simulink model "RL_sus_quarter_sim"  (R2025a)
settings: Solver=FixedStepAuto  StartTime=0.0  StopTime=20  FixedStep=0.001  RelTol=1e-3
model workspace (MAT data in the model file):
  G0 : Simulink.Parameter (value not decoded)
  Q_F : Simulink.Parameter (value not decoded)
  Q_dot_s : Simulink.Parameter (value not decoded)
  Q_dot_s_h : Simulink.Parameter (value not decoded)
  Q_dot_u : Simulink.Parameter (value not decoded)
  Q_flec : Simulink.Parameter (value not decoded)
  Q_flec_t : Simulink.Parameter (value not decoded)
  b_deflec : Simulink.Parameter (value not decoded)
  bump_height : Simulink.Parameter (value not decoded)
  bump_lenth : Simulink.Parameter (value not decoded)
  bump_start : Simulink.Parameter (value not decoded)
  f0 : Simulink.Parameter (value not decoded)
  kt : Simulink.Parameter (value not decoded)
  ms : Simulink.Parameter (value not decoded)
  n0 : Simulink.Parameter (value not decoded)
  n1 : Simulink.Parameter (value not decoded)
  omega_1 : Simulink.Parameter (value not decoded)
  omega_2 : Simulink.Parameter (value not decoded)
  omega_3 : Simulink.Parameter (value not decoded)
  omega_4 : Simulink.Parameter (value not decoded)
  ramp_height : Simulink.Parameter (value not decoded)
  ramp_lenth : Simulink.Parameter (value not decoded)
  ramp_start : Simulink.Parameter (value not decoded)
  sine_amp : Simulink.Parameter (value not decoded)
  sine_freq : Simulink.Parameter (value not decoded)
  u : Simulink.Parameter (value not decoded)
symbols that are objects in the model workspace (value not decoded): b_deflec, bump_height, bump_lenth, bump_start, f0, G0, kt, ms, n0, n1, omega_1, omega_2, omega_3, omega_4, Q_dot_s, Q_dot_s_h, Q_F, Q_flec, Q_flec_t, ramp_height, ramp_lenth, ramp_start, sine_amp, sine_freq
undefined symbols (not defined in the file): Ground, Hook, SH_ADD_new_as_as_xdef
libraries: fl_lib x250, nesl_utility x48, sharedTrackingLibrary x34, dspstat3 x18, simulink x3, deeplib x2, slpidlib x1
(part 5 of 12)

== system RL_sus_quarter_sim/Quarter_sys/Control/Y_1/SH_ADD_new_xdef_vs ==
  x_def : Inport
  v_def : Inport  Port=2
  v_s : Inport  Port=3
  a_s : Inport  Port=4
  a_def : Inport  Port=5
  2nd_FS_adef_vs : Subsystem
  ADD : Subsystem
  SH : Subsystem
  Scope : Scope
      settings: ActiveDisplayYMinimum=-69.71709  ActiveDisplayYMaximum=42.91727  DataLoggingVariableName=ScopeData19
  Scope1 : Scope
      settings: ActiveDisplayYMinimum=-36.33724  ActiveDisplayYMaximum=1.39762  DataLoggingVariableName=ScopeData21
  Switch1 : Switch  Criteria=u2 > Threshold  SaturateOnIntegerOverflow=off  InputSameDT=off
  F_sus : Outport
  wires:
  v_def/1 -> ADD/2(v_def), SH/1(v_def)
  x_def/1 -> Scope1/1, SH/3(x_def), ADD/1(x_def)
  ADD/1(F_sus1) -> Switch1/1
  SH/1(Out1) -> Switch1/3
  v_s/1 -> 2nd_FS_adef_vs/1(vs), SH/2(v_s)
  a_s/1 -> ADD/3(a_s)
  2nd_FS_adef_vs/1(FS2) -> Scope/1, Switch1/2
  Switch1/1 -> F_sus/1
  a_def/1 -> 2nd_FS_adef_vs/2(adef)

== system RL_sus_quarter_sim/Quarter_sys/Control/Y_1/Sky-Hook ==
  v_def : Inport
  v_s : Inport  Port=2
  x_def : Inport  Port=3
  Add : Sum
  Add1 : Sum
  Constant : Constant  Value=-1
  Constant1 : Constant
  Delta_C : Gain  Gain=500
  Gain : Gain  Gain=-1
  Lmbada_C : Constant  Value=1000
  Product : Product
  Product1 : Product
  Switch : Switch  Criteria=u2 > Threshold  SaturateOnIntegerOverflow=off  InputSameDT=off
  ks : Gain  Gain=-20000
  F_sus : Outport
  wires:
  Product/1 -> Switch/2
  v_s/1 -> Product/2
  v_def/1 -> Product1/1, Product/1
  Add/1 -> Product1/2
  Switch/1 -> Delta_C/1
  Product1/1 -> Gain/1
  Constant/1 -> Switch/3
  Constant1/1 -> Switch/1
  Lmbada_C/1 -> Add/2
  Delta_C/1 -> Add/1
  Gain/1 -> Add1/1
  Add1/1 -> F_sus/1
  ks/1 -> Add1/2
  x_def/1 -> ks/1

== system RL_sus_quarter_sim/Quarter_sys/Control/Y_1/decouple_Hinf ==
  x_def : Inport
  v_s : Inport  Port=2
  v_def : Inport  Port=3
  a_def : Inport  Port=4
  a_s : Inport  Port=5
  a_u : Inport  Port=6
  v_u : Inport  Port=7
  x_s : Inport  Port=8
  Add : Sum  Inputs=+-
  Add1 : Sum  Inputs=--
  Add2 : Sum
  Add3 : Sum
  Constant : Constant  Value=[10,10]  VectorParams1D=off
  Gain : Gain  Gain=-1
  Gain1 : Gain  Gain=20000
  Gain2 : Gain  Gain=1500
  Mux : Mux  Inputs=2
  Product : Product  Multiplication=Matrix(*)
  cs : Gain  Gain=-1000
  ks : Gain  Gain=-20000
  ms : Gain  Gain=400
  F_sus : Outport
  wires:
  Add1/1 -> Add/2  "alpha"
  Add/1 -> Add3/1
  Gain/1 -> ms/1  "v"
  Gain1/1 -> Add1/1
  Gain2/1 -> Add1/2
  ms/1 -> Add/1
  Add2/1 -> Add3/2  "passive"
  ks/1 -> Add2/1
  x_def/1 -> Mux/1, ks/1, Gain1/1
  v_def/1 -> cs/1, Gain2/1, Mux/2
  cs/1 -> Add2/2
  Add3/1 -> F_sus/1
  Constant/1 -> Product/1
  Product/1 -> Gain/1
  Mux/1 -> Product/2

== system RL_sus_quarter_sim/Quarter_sys/Control/Y_1/decouple_simple ==
  x_def : Inport
  v_s : Inport  Port=2
  v_def : Inport  Port=3
  a_def : Inport  Port=4
  a_s : Inport  Port=5
  a_u : Inport  Port=6
  v_u : Inport  Port=7
  x_s : Inport  Port=8
  x_u : Inport  Port=9
  Add : Sum  Inputs=+-
  Add1 : Sum  Inputs=--
  Add2 : Sum
  Add3 : Sum
  Gain1 : Gain  Gain=20000
  Gain2 : Gain  Gain=1500
  Gain3 : Gain  Gain=(-kt+100)/ms
  Gain4 : Gain  Gain=10/ms
  ms : Gain  Gain=400
  passive : Subsystem
  F_sus : Outport
  wires:
  Add3/1 -> F_sus/1
  v_def/1 -> passive/2(In2), Gain2/1  "vdef"
  x_def/1 -> Gain1/1, passive/1(In1)  "xdef"
  ms/1 -> Add/1
  Gain2/1 -> Add1/2
  Gain1/1 -> Add1/1
  Add2/1 -> ms/1  "v"
  Add/1 -> Add3/1
  Add1/1 -> Add/2  "alpha"
  passive/1(passive) -> Add3/2
  x_u/1 -> Gain3/1
  v_u/1 -> Gain4/1
  Gain3/1 -> Add2/1
  Gain4/1 -> Add2/2

== system RL_sus_quarter_sim/Quarter_sys/Control/Y_1/freq semi ==
  x_def : Inport
  v_def : Inport  Port=2
  a_def : Inport  Port=3
  a_s : Inport  Port=4
  v_s : Inport  Port=5
  a_u : Inport  Port=6
  ADD : Subsystem
  Multiport Switch : MultiPortSwitch  SaturateOnIntegerOverflow=off  InputSameDT=off
  Multiport Switch1 : MultiPortSwitch  Commented=on  SaturateOnIntegerOverflow=off  InputSameDT=off
  SH : Subsystem
  Scope : Scope
      settings: ActiveDisplayYMinimum=1.00019  ActiveDisplayYMaximum=3.05477  DataLoggingVariableName=ScopeData6
  Scope1 : Scope  Commented=on  NumInputPorts=2
      settings: ActiveDisplayYMinimum=-22.33402  ActiveDisplayYMaximum=17.66511  DataLoggingVariableName=ScopeData5
  Scope2 : Scope  Commented=on
      settings: ActiveDisplayYMinimum=-1695.55215  ActiveDisplayYMaximum=1442.87782  DataLoggingVariableName=ScopeData6
  Scope3 : Scope  Commented=on
      settings: ActiveDisplayYMinimum=-838.91856  ActiveDisplayYMaximum=95.65649  DataLoggingVariableName=ScopeData7
  Subsystem : Subsystem
  Subsystem1 : Subsystem
  Subsystem2 : Subsystem  Commented=on
  Subsystem3 : Subsystem  Commented=on
  Switch : Switch  Commented=on  Criteria=u2 > Threshold  SaturateOnIntegerOverflow=off  InputSameDT=off
  To Workspace : ToWorkspace  VariableName=FS_result  SampleTime=-1
  F_sus : Outport
  wires:
  v_s/1 -> Subsystem/1(vs), SH/2(v_s)
  a_s/1 -> ADD/3(a_s), Subsystem/3(as)
  v_def/1 -> ADD/2(v_def), SH/1(v_def), Subsystem1/1(v_def), Subsystem2/1(v_def), Subsystem3/1(v_def)
  x_def/1 -> Subsystem2/2(x_def), Subsystem3/2(x_def), Subsystem1/2(x_def), SH/3(x_def), ADD/1(x_def)
  Subsystem1/1(Out1) -> Multiport Switch1/4, Switch/1, Multiport Switch/4
  SH/1(Out1) -> Multiport Switch/2
  ADD/1(F_sus1) -> Multiport Switch/3
  Multiport Switch/1 -> F_sus/1
  Multiport Switch1/1 -> ?
  Subsystem2/1(Out1) -> Multiport Switch1/2, Switch/3
  Subsystem3/1(Out1) -> Multiport Switch1/3
  Switch/1 -> Scope2/1
  Subsystem/2(FS_1) -> Scope1/1, Scope3/1, Switch/2
  a_u/1 -> Subsystem/2(au)
  Subsystem/3(FS_2) -> Scope1/2
  Subsystem/1(Select) -> Multiport Switch1/1, Scope/1, To Workspace/1, Multiport Switch/1

== system RL_sus_quarter_sim/Quarter_sys/Control/Y_1/imp_force_RL_model ==
  x_def : Inport
  v_s : Inport  Port=2
  v_def : Inport  Port=3
  a_def : Inport  Port=4
  a_s : Inport  Port=5
  Add2 : Sum  Inputs=+++
  Add3 : Sum
  Gain : Gain  Gain=1000
  Gain1 : Gain  Gain=1/5
  Gain2 : Gain  Gain=1/0.3
  Gain3 : Gain  Gain=1/0.03
  Mux : Mux
  Predict1 : deeplib/Predict  Network=Network from MAT-file  NetworkFunction=squeezenet  NetworkFilePath=D:\Project\GOPS\mdl\RL_model\TD3_270374_opt.mat  MiniBatchSize=128  InputDataFormats={ 'input_1', 'UU' }  Predictions=on  Activations={}  ForceInterpretedSim=off  EnableDLNetwork=on  LastKnownNetworkFilePath='D:\Project\GOPS\mdl\RL_model\TD3_270374_opt.mat'  LastKnownNetworkTimeStamp=739967.681944444426335394382476806640625
  Rate Transition : RateTransition  OutPortSampleTime=0.01
  Reshape : Reshape  OutputDimensionality=Row vector (2-D)
  Reshape2 : Reshape
  Saturation : Saturate  UpperLimit=1000  LowerLimit=-1000
  Subsystem : Subsystem
  bkkcc : Subsystem
  cs1 : Gain  Gain=-1000
  ks1 : Gain  Gain=-20000
  F_sus : Outport
  F_ctr : Outport  Port=2
  wires:
  Gain2/1 -> Mux/4
  Rate Transition/1 -> Predict1/1
  Reshape2/1 -> Gain/1
  Gain/1 -> Saturation/1
  Gain3/1 -> Mux/3
  Gain1/1 -> Mux/1
  Reshape/1 -> Rate Transition/1
  Mux/1 -> Reshape/1
  Predict1/1 -> Reshape2/1
  v_def/1 -> bkkcc/1(v_def), cs1/1, Gain2/1
  a_def/1 -> bkkcc/3(a_def)
  cs1/1 -> Add2/2  "F_damper"
  ks1/1 -> Add2/1
  x_def/1 -> ks1/1, bkkcc/2(x_def), Gain3/1
  Subsystem/1(Out1) -> bkkcc/4(param_ctr)
  bkkcc/1(F_bkkcc) -> Add2/3
  v_s/1 -> Subsystem/1(v_s), Mux/2
  Add2/1 -> Add3/2
  Add3/1 -> F_sus/1
  a_s/1 -> Gain1/1
  Saturation/1 -> Add3/1, F_ctr/1

== system RL_sus_quarter_sim/Quarter_sys/Control/Y_1/lqr ==
  x_s : Inport
  v_s : Inport  Port=2
  x_def : Inport  Port=3
  v_def : Inport  Port=4
  Add : Sum  Inputs=+-
  Add1 : Sum  Inputs=+++
  Add2 : Sum  Inputs=+-
  Gain : Gain  Gain=-1
  K : Constant  Value="[-824.335747522357\t31.6227766016762\t-0.106412814889091\t-3.16537773169978]"
  Mux : Mux
  Product : Product  Multiplication=Matrix(*)
  To Workspace : ToWorkspace  VariableName=F_if_imp  SampleTime=-1
  cs : Gain  Gain=-1000
  ks : Gain  Gain=-20000
  F_sus : Outport
  wires:
  v_def/1 -> Add2/2, cs/1
  v_s/1 -> Add2/1, Mux/2  "vs"
  x_s/1 -> Add/1, ks/1, Mux/1  "xs"
  Add1/1 -> F_sus/1
  ks/1 -> Add1/1
  cs/1 -> Add1/2  "F_damper"
  x_def/1 -> Add/2
  Add/1 -> Mux/3  "xu"
  Add2/1 -> Mux/4  "vu"
  K/1 -> Product/2
  Mux/1 -> Product/1
  Product/1 -> Gain/1
  Gain/1 -> Add1/3, To Workspace/1

== system RL_sus_quarter_sim/Quarter_sys/Passive/Y_1/P_0 ==
  x_def : Inport
  v_def : Inport  Port=2
  a_def : Inport  Port=3
  Add1 : Sum
  Ideal Force Sensor : fl_lib/Mechanical/Mechanical Sensors/Ideal Force Sensor
  Ideal Translational Velocity Source : fl_lib/Mechanical/Mechanical Sources/Ideal Translational Velocity Source
  Mechanical Translational Reference : fl_lib/Mechanical/Translational Elements/Mechanical Translational Reference
  Mechanical Translational Reference1 : fl_lib/Mechanical/Translational Elements/Mechanical Translational Reference
  PS-Simulink Converter : nesl_utility/PS-Simulink Converter  PhysicalDomain=network_engine_domain  SubClassName=ps_output  LeftPortType=input  RightPortType=output  PseudoPeriodic=off  Frequencies=[]  VectorFormat=inherit  Unit=inherit  AffineConversion=off
  Scope : Scope  NumInputPorts=2
      settings: ActiveDisplayYMinimum=-2784.63973  ActiveDisplayYMaximum=3155.95467
  Simulink-PS Converter : nesl_utility/Simulink-PS Converter  PhysicalDomain=network_engine_domain  SubClassName=ps_input  LeftPortType=input  RightPortType=output  PseudoPeriodic=off  Frequencies=[]  NoiseDistribution=none  NoiseParameters=[]  Unit=1  AffineConversion=off  FilteringAndDerivatives=provide  SimscapeFilterOrder=1  InputFilterTimeConstant=0.001  UdotUserProvided=0
  Solver Configuration : nesl_utility/Solver Configuration  PhysicalDomain=network_engine_domain  SubClassName=solver  LeftPortType=input  RightPortType=generic  Tones=[]  Harmonics=[]  SimulateNoise=off  Profile=off  UseLocalSampling=off  EnableSwitchedLinearOptims=on  FrequencyDomain=off  UseCCode=off  RelTol=0.001  AbsTol=0.001  MinStep=1e-09  ToWorkspace=off  RevertToSquareIcSolve=off  NumHomotopyIterations=100  PhasorMode=off  PhasorModeNumHarmonics=1  ConsistencySolver=NEWTON_XTOL_AFTER_FTOL  IndexReductionMethod=DerivativeReplacement  DoDC=off  ResidualTolerance=1e-09  ConsistencyTolSource=GLOBAL  ConsistencyAbsTol=0.001  ConsistencyRelTol=0.001  ConsistencyTolFactor=0.001  UseLocalSolver=off  LocalSolverChoice=NE_BACKWARD_EULER_ADVANCER  ResolveIndetEquations=on  FunctionEvalNumThread=1  LocalSolverSampleTime=0.001  DoFixedCost=off  MaxNonlinIter=3  MaxModeIter=2  ComputeImpulses=off  ImpulseIterations=2  LinearAlgebra=auto  LinearAlgebraNumThread=0  EquationFormulation=NE_TIME_EF  DelaysMemoryBudget=1024  AutomaticFiltering=on  FilteringTimeConstant=0.001  PartitionStorageMethod=AS_NEEDED  PartitionMemoryBudget=1024  PartitionMethod=ROBUST  MultibodyUseLocalSolver=off  MultibodyLocalSolverChoice=ODE1  MultibodyLocalSolverSampleTime=0.001
  Subsystem : Subsystem  Variant=on  VariantControlMode=label  VariantControl=Subsystem  LabelModeActiveChoice=p0_k6
  cs : Gain  Gain=-2000
  ks : Gain  Gain=-200000
  F_sus : Outport
  wires:
  x_def/1 -> ks/1
  cs/1 -> Add1/2
  ks/1 -> Add1/1
  v_def/1 -> Simulink-PS Converter/1, cs/1
  PS-Simulink Converter/1 -> F_sus/1, Scope/1
  connections:
  Mechanical Translational Reference1/LConn1 -- Solver Configuration/RConn1 -- Ideal Translational Velocity Source/LConn1
  Simulink-PS Converter/RConn1 -- Ideal Translational Velocity Source/RConn1
  Ideal Force Sensor/RConn1 -- Mechanical Translational Reference/LConn1
  PS-Simulink Converter/LConn1 -- Ideal Force Sensor/RConn2
  Subsystem/LConn1 -- Ideal Translational Velocity Source/RConn2
  Subsystem/RConn1 -- Ideal Force Sensor/LConn1

== system RL_sus_quarter_sim/Quarter_sys/Passive/Y_1/P_1 ==
  x_def : Inport
  v_def : Inport  Port=2
  a_def : Inport  Port=3
  Add1 : Sum
  Ideal Force Sensor : fl_lib/Mechanical/Mechanical Sensors/Ideal Force Sensor
  Ideal Translational Velocity Source : fl_lib/Mechanical/Mechanical Sources/Ideal Translational Velocity Source
  Mechanical Translational Reference : fl_lib/Mechanical/Translational Elements/Mechanical Translational Reference
  Mechanical Translational Reference1 : fl_lib/Mechanical/Translational Elements/Mechanical Translational Reference
  PS-Simulink Converter : nesl_utility/PS-Simulink Converter  PhysicalDomain=network_engine_domain  SubClassName=ps_output  LeftPortType=input  RightPortType=output  PseudoPeriodic=off  Frequencies=[]  VectorFormat=inherit  Unit=inherit  AffineConversion=off
  Scope : Scope  NumInputPorts=2
      settings: ActiveDisplayYMinimum=-2784.63973  ActiveDisplayYMaximum=3155.95467
  Simulink-PS Converter : nesl_utility/Simulink-PS Converter  PhysicalDomain=network_engine_domain  SubClassName=ps_input  LeftPortType=input  RightPortType=output  PseudoPeriodic=off  Frequencies=[]  NoiseDistribution=none  NoiseParameters=[]  Unit=1  AffineConversion=off  FilteringAndDerivatives=provide  SimscapeFilterOrder=1  InputFilterTimeConstant=0.001  UdotUserProvided=1
  Solver Configuration : nesl_utility/Solver Configuration  PhysicalDomain=network_engine_domain  SubClassName=solver  LeftPortType=input  RightPortType=generic  Tones=[]  Harmonics=[]  SimulateNoise=off  Profile=off  UseLocalSampling=off  EnableSwitchedLinearOptims=on  FrequencyDomain=off  UseCCode=off  RelTol=0.001  AbsTol=0.001  MinStep=1e-09  ToWorkspace=off  RevertToSquareIcSolve=off  NumHomotopyIterations=100  PhasorMode=off  PhasorModeNumHarmonics=1  ConsistencySolver=NEWTON_XTOL_AFTER_FTOL  IndexReductionMethod=DerivativeReplacement  DoDC=off  ResidualTolerance=1e-09  ConsistencyTolSource=GLOBAL  ConsistencyAbsTol=0.001  ConsistencyRelTol=0.001  ConsistencyTolFactor=0.001  UseLocalSolver=off  LocalSolverChoice=NE_BACKWARD_EULER_ADVANCER  ResolveIndetEquations=on  FunctionEvalNumThread=1  LocalSolverSampleTime=0.001  DoFixedCost=off  MaxNonlinIter=3  MaxModeIter=2  ComputeImpulses=off  ImpulseIterations=2  LinearAlgebra=auto  LinearAlgebraNumThread=0  EquationFormulation=NE_TIME_EF  DelaysMemoryBudget=1024  AutomaticFiltering=on  FilteringTimeConstant=0.001  PartitionStorageMethod=AS_NEEDED  PartitionMemoryBudget=1024  PartitionMethod=ROBUST  MultibodyUseLocalSolver=off  MultibodyLocalSolverChoice=ODE1  MultibodyLocalSolverSampleTime=0.001
  Subsystem : Subsystem  Variant=on  VariantControlMode=label  VariantControl=Subsystem  LabelModeActiveChoice=p1_k3
  cs : Gain  Gain=-2000
  ks : Gain  Gain=-200000
  F_sus : Outport
  wires:
  PS-Simulink Converter/1 -> F_sus/1, Scope/1
  v_def/1 -> cs/1, Simulink-PS Converter/1
  ks/1 -> Add1/1
  cs/1 -> Add1/2
  x_def/1 -> ks/1
  a_def/1 -> Simulink-PS Converter/2
  connections:
  Subsystem/RConn1 -- Ideal Force Sensor/LConn1
  Subsystem/LConn1 -- Ideal Translational Velocity Source/RConn2
  PS-Simulink Converter/LConn1 -- Ideal Force Sensor/RConn2
  Ideal Force Sensor/RConn1 -- Mechanical Translational Reference/LConn1
  Simulink-PS Converter/RConn1 -- Ideal Translational Velocity Source/RConn1
  Solver Configuration/RConn1 -- Mechanical Translational Reference1/LConn1 -- Ideal Translational Velocity Source/LConn1

== system RL_sus_quarter_sim/Quarter_sys/Passive/Y_1/P_test ==
  x_def : Inport
  v_def : Inport  Port=2
  a_def : Inport  Port=3
  Add : Sum  Inputs=+-
  Add1 : Sum
  Ideal Force Sensor : fl_lib/Mechanical/Mechanical Sensors/Ideal Force Sensor
  Ideal Translational Velocity Source : fl_lib/Mechanical/Mechanical Sources/Ideal Translational Velocity Source
  Integrator : Integrator
  Mechanical Translational Reference : fl_lib/Mechanical/Translational Elements/Mechanical Translational Reference
  Mechanical Translational Reference1 : fl_lib/Mechanical/Translational Elements/Mechanical Translational Reference
  PS-Simulink Converter : nesl_utility/PS-Simulink Converter  PhysicalDomain=network_engine_domain  SubClassName=ps_output  LeftPortType=input  RightPortType=output  PseudoPeriodic=off  Frequencies=[]  VectorFormat=inherit  Unit=inherit  AffineConversion=off
  Scope : Scope  NumInputPorts=2
      settings: ActiveDisplayYMinimum=-1294.98501  ActiveDisplayYMaximum=1379.176
  Simulink-PS Converter : nesl_utility/Simulink-PS Converter  PhysicalDomain=network_engine_domain  SubClassName=ps_input  LeftPortType=input  RightPortType=output  PseudoPeriodic=off  Frequencies=[]  NoiseDistribution=none  NoiseParameters=[]  Unit=1  AffineConversion=off  FilteringAndDerivatives=provide  SimscapeFilterOrder=1  InputFilterTimeConstant=0.001  UdotUserProvided=1
  Solver Configuration : nesl_utility/Solver Configuration  PhysicalDomain=network_engine_domain  SubClassName=solver  LeftPortType=input  RightPortType=generic  Tones=[]  Harmonics=[]  SimulateNoise=off  Profile=off  UseLocalSampling=off  EnableSwitchedLinearOptims=on  FrequencyDomain=off  UseCCode=off  RelTol=0.001  AbsTol=0.001  MinStep=1e-09  ToWorkspace=off  RevertToSquareIcSolve=off  NumHomotopyIterations=100  PhasorMode=off  PhasorModeNumHarmonics=1  ConsistencySolver=NEWTON_XTOL_AFTER_FTOL  IndexReductionMethod=DerivativeReplacement  DoDC=off  ResidualTolerance=1e-09  ConsistencyTolSource=GLOBAL  ConsistencyAbsTol=0.001  ConsistencyRelTol=0.001  ConsistencyTolFactor=0.001  UseLocalSolver=off  LocalSolverChoice=NE_BACKWARD_EULER_ADVANCER  ResolveIndetEquations=on  FunctionEvalNumThread=1  LocalSolverSampleTime=0.001  DoFixedCost=off  MaxNonlinIter=3  MaxModeIter=2  ComputeImpulses=off  ImpulseIterations=2  LinearAlgebra=auto  LinearAlgebraNumThread=0  EquationFormulation=NE_TIME_EF  DelaysMemoryBudget=1024  AutomaticFiltering=on  FilteringTimeConstant=0.001  PartitionStorageMethod=AS_NEEDED  PartitionMemoryBudget=1024  PartitionMethod=ROBUST  MultibodyUseLocalSolver=off  MultibodyLocalSolverChoice=ODE1  MultibodyLocalSolverSampleTime=0.001
  Subsystem : Subsystem  Commented=on  Variant=on  VariantControlMode=label  VariantControl=Subsystem  LabelModeActiveChoice=p1_k3
  Translational Damper : fl_lib/Mechanical/Translational Elements/Translational Damper  D=2000 N*s/m  v_specify=off  v_priority=None  v=0 m/s  v_nominal_specify=off  v_nominal_value=1  v_nominal_unit=m/s  f_specify=off  f_priority=None  f=0 N  f_nominal_specify=off  f_nominal_value=1  f_nominal_unit=N
  Translational Spring1 : fl_lib/Mechanical/Translational Elements/Translational Spring  spr_rate=200000 N/m  v_specify=off  v_priority=None  v=0 m/s  v_nominal_specify=off  v_nominal_value=1  v_nominal_unit=m/s  f_specify=off  f_priority=None  f=0 N  f_nominal_specify=off  f_nominal_value=1  f_nominal_unit=N  x_specify=off  x_priority=High  x=0 m  x_nominal_specify=off  x_nominal_value=1  x_nominal_unit=m
  Translational Spring2 : fl_lib/Mechanical/Translational Elements/Translational Spring  spr_rate=20000 N/m  v_specify=off  v_priority=None  v=0 m/s  v_nominal_specify=off  v_nominal_value=1  v_nominal_unit=m/s  f_specify=off  f_priority=None  f=0 N  f_nominal_specify=off  f_nominal_value=1  f_nominal_unit=N  x_specify=off  x_priority=High  x=0 m  x_nominal_specify=off  x_nominal_value=1  x_nominal_unit=m
  cs : Gain  Gain=-2000
  cs1 : Gain  Gain=20000/2000
  ks : Gain  Gain=-20000
  ks1 : Gain  Gain=-20000
  F_sus : Outport
  wires:
  a_def/1 -> Simulink-PS Converter/2
  x_def/1 -> ks/1
  cs/1 -> Add1/2
  ks/1 -> Add1/1
  v_def/1 -> ks1/1, Simulink-PS Converter/1, cs/1
  PS-Simulink Converter/1 -> Scope/1, F_sus/1
  Integrator/1 -> cs1/1, Scope/2
  ks1/1 -> Add/1
  Add/1 -> Integrator/1
  cs1/1 -> Add/2
  connections:
  Ideal Translational Velocity Source/LConn1 -- Mechanical Translational Reference1/LConn1 -- Solver Configuration/RConn1
  Simulink-PS Converter/RConn1 -- Ideal Translational Velocity Source/RConn1
  Ideal Force Sensor/RConn1 -- Mechanical Translational Reference/LConn1
  PS-Simulink Converter/LConn1 -- Ideal Force Sensor/RConn2
  Subsystem/LConn1 -- Translational Spring2/LConn1 -- Translational Damper/LConn1 -- Ideal Translational Velocity Source/RConn2
  Subsystem/RConn1 -- Translational Spring2/RConn1 -- Translational Spring1/RConn1 -- Ideal Force Sensor/LConn1
  Translational Spring1/LConn1 -- Translational Damper/RConn1

== system RL_sus_quarter_sim/Quarter_sys/Passive/Y_1/Passive ==
  x_def : Inport
  v_def : Inport  Port=2
  a_def : Inport  Port=3
  Add1 : Sum
  cs : Gain  Gain=-7.5
  ks : Gain  Gain=-900
  F_sus : Outport
  wires:
  Add1/1 -> F_sus/1
  v_def/1 -> cs/1
  ks/1 -> Add1/1
  cs/1 -> Add1/2
  x_def/1 -> ks/1

== system RL_sus_quarter_sim/Quarter_sys/Passive/Y_1/Sky-Hook ==
  x_def : Inport
  v_def : Inport  Port=2
  a_def : Inport  Port=3
  Add : Sum  Inputs=+-
  Add1 : Sum
  Ideal Force Sensor : fl_lib/Mechanical/Mechanical Sensors/Ideal Force Sensor
  Ideal Translational Velocity Source : fl_lib/Mechanical/Mechanical Sources/Ideal Translational Velocity Source
  Integrator : Integrator
  Mechanical Translational Reference : fl_lib/Mechanical/Translational Elements/Mechanical Translational Reference
  Mechanical Translational Reference1 : fl_lib/Mechanical/Translational Elements/Mechanical Translational Reference
  PS-Simulink Converter : nesl_utility/PS-Simulink Converter  PhysicalDomain=network_engine_domain  SubClassName=ps_output  LeftPortType=input  RightPortType=output  PseudoPeriodic=off  Frequencies=[]  VectorFormat=inherit  Unit=inherit  AffineConversion=off
  Scope : Scope  NumInputPorts=2
      settings: ActiveDisplayYMinimum=-1294.98501  ActiveDisplayYMaximum=1379.176
  Simulink-PS Converter : nesl_utility/Simulink-PS Converter  PhysicalDomain=network_engine_domain  SubClassName=ps_input  LeftPortType=input  RightPortType=output  PseudoPeriodic=off  Frequencies=[]  NoiseDistribution=none  NoiseParameters=[]  Unit=1  AffineConversion=off  FilteringAndDerivatives=provide  SimscapeFilterOrder=1  InputFilterTimeConstant=0.001  UdotUserProvided=1
  Solver Configuration : nesl_utility/Solver Configuration  PhysicalDomain=network_engine_domain  SubClassName=solver  LeftPortType=input  RightPortType=generic  Tones=[]  Harmonics=[]  SimulateNoise=off  Profile=off  UseLocalSampling=off  EnableSwitchedLinearOptims=on  FrequencyDomain=off  UseCCode=off  RelTol=0.001  AbsTol=0.001  MinStep=1e-09  ToWorkspace=off  RevertToSquareIcSolve=off  NumHomotopyIterations=100  PhasorMode=off  PhasorModeNumHarmonics=1  ConsistencySolver=NEWTON_XTOL_AFTER_FTOL  IndexReductionMethod=DerivativeReplacement  DoDC=off  ResidualTolerance=1e-09  ConsistencyTolSource=GLOBAL  ConsistencyAbsTol=0.001  ConsistencyRelTol=0.001  ConsistencyTolFactor=0.001  UseLocalSolver=off  LocalSolverChoice=NE_BACKWARD_EULER_ADVANCER  ResolveIndetEquations=on  FunctionEvalNumThread=1  LocalSolverSampleTime=0.001  DoFixedCost=off  MaxNonlinIter=3  MaxModeIter=2  ComputeImpulses=off  ImpulseIterations=2  LinearAlgebra=auto  LinearAlgebraNumThread=0  EquationFormulation=NE_TIME_EF  DelaysMemoryBudget=1024  AutomaticFiltering=on  FilteringTimeConstant=0.001  PartitionStorageMethod=AS_NEEDED  PartitionMemoryBudget=1024  PartitionMethod=ROBUST  MultibodyUseLocalSolver=off  MultibodyLocalSolverChoice=ODE1  MultibodyLocalSolverSampleTime=0.001
  Subsystem : Subsystem  Commented=on  Variant=on  VariantControlMode=label  VariantControl=Subsystem  LabelModeActiveChoice=p1_k3
  Translational Damper : fl_lib/Mechanical/Translational Elements/Translational Damper  D=2000 N*s/m  v_specify=off  v_priority=None  v=0 m/s  v_nominal_specify=off  v_nominal_value=1  v_nominal_unit=m/s  f_specify=off  f_priority=None  f=0 N  f_nominal_specify=off  f_nominal_value=1  f_nominal_unit=N
  Translational Spring1 : fl_lib/Mechanical/Translational Elements/Translational Spring  spr_rate=200000 N/m  v_specify=off  v_priority=None  v=0 m/s  v_nominal_specify=off  v_nominal_value=1  v_nominal_unit=m/s  f_specify=off  f_priority=None  f=0 N  f_nominal_specify=off  f_nominal_value=1  f_nominal_unit=N  x_specify=off  x_priority=High  x=0 m  x_nominal_specify=off  x_nominal_value=1  x_nominal_unit=m
  Translational Spring2 : fl_lib/Mechanical/Translational Elements/Translational Spring  spr_rate=20000 N/m  v_specify=off  v_priority=None  v=0 m/s  v_nominal_specify=off  v_nominal_value=1  v_nominal_unit=m/s  f_specify=off  f_priority=None  f=0 N  f_nominal_specify=off  f_nominal_value=1  f_nominal_unit=N  x_specify=off  x_priority=High  x=0 m  x_nominal_specify=off  x_nominal_value=1  x_nominal_unit=m
  cs : Gain  Gain=-2000
  cs1 : Gain  Gain=20000/2000
  ks : Gain  Gain=-20000
  ks1 : Gain  Gain=-20000
  F_sus : Outport
  wires:
  cs1/1 -> Add/2
  Add/1 -> Integrator/1
  ks1/1 -> Add/1
  Integrator/1 -> Scope/2, cs1/1
  PS-Simulink Converter/1 -> F_sus/1, Scope/1
  v_def/1 -> cs/1, Simulink-PS Converter/1, ks1/1
  ks/1 -> Add1/1
  cs/1 -> Add1/2
  x_def/1 -> ks/1
  a_def/1 -> Simulink-PS Converter/2
  connections:
  Translational Spring1/LConn1 -- Translational Damper/RConn1
  Translational Spring2/RConn1 -- Translational Spring1/RConn1 -- Subsystem/RConn1 -- Ideal Force Sensor/LConn1
  Translational Spring2/LConn1 -- Translational Damper/LConn1 -- Subsystem/LConn1 -- Ideal Translational Velocity Source/RConn2
  PS-Simulink Converter/LConn1 -- Ideal Force Sensor/RConn2
  Ideal Force Sensor/RConn1 -- Mechanical Translational Reference/LConn1
  Simulink-PS Converter/RConn1 -- Ideal Translational Velocity Source/RConn1
  Solver Configuration/RConn1 -- Mechanical Translational Reference1/LConn1 -- Ideal Translational Velocity Source/LConn1

== system RL_sus_quarter_sim/road_profile/origin/road_profile/Bump ==
  Add : Sum
  Add1 : Sum  Inputs=+-
  Clock1 : Clock
  Constant : Constant  Value=bump_height
  Constant1 : Constant  Value=0
  Constant2 : Constant  Value=u
  Constant3 : Constant  Value=bump_start
  Constant4 : Constant  Value=bump_lenth
  Divide : Product  Inputs=*/
  Gain : Gain  Gain=1/3.6
  Product : Product
  Sine Wave1 : Sin  TimeSource=Use external signal  Amplitude=bump_height  Frequency=2*pi*1  Phase=-1/2*pi  SampleTime=0
  Switch : Switch  Criteria=u2 > Threshold  Threshold=bump_start  SaturateOnIntegerOverflow=off  InputSameDT=off
  Switch1 : Switch  Criteria=u2 > Threshold  Threshold=bump_lenth+bump_start  SaturateOnIntegerOverflow=off  InputSameDT=off
  Zr : Outport  VectorParamsAs1DForOutWhenUnconnected=off
  wires:
  Divide/1 -> Sine Wave1/1
  Constant/1 -> Add/2
  Add/1 -> Switch/1
  Constant4/1 -> Divide/2
  Add1/1 -> Divide/1
  Product/1 -> Gain/1
  Constant2/1 -> Product/1
  Constant3/1 -> Add1/2
  Constant1/1 -> Switch1/1, Switch/3
  Switch/1 -> Switch1/3
  Gain/1 -> Switch1/2, Switch/2, Add1/1
  Sine Wave1/1 -> Add/1
  Clock1/1 -> Product/2
  Switch1/1 -> Zr/1

== system RL_sus_quarter_sim/road_profile/origin/road_profile/Ramp ==
  Add : Sum
  Add1 : Sum  Inputs=+-
  Clock1 : Clock
  Constant : Constant  Value=ramp_height
  Constant1 : Constant  Value=0
  Constant2 : Constant  Value=u
  Constant3 : Constant  Value=ramp_start
  Constant4 : Constant  Value=ramp_lenth
  Constant5 : Constant  Value=ramp_height
  Divide : Product  Inputs=*/
  Gain : Gain  Gain=1/3.6
  Gain1 : Gain  Gain=2
  Gain2 : Gain  Gain=1/2
  Product : Product
  Sine Wave1 : Sin  TimeSource=Use external signal  Amplitude=bump_height/2  Frequency=2*pi*1  Phase=-1/2*pi  SampleTime=0
  Switch : Switch  Criteria=u2 > Threshold  Threshold=bump_start  SaturateOnIntegerOverflow=off  InputSameDT=off
  Switch1 : Switch  Criteria=u2 > Threshold  Threshold=ramp_lenth+ramp_start  SaturateOnIntegerOverflow=off  InputSameDT=off
  Zr : Outport  VectorParamsAs1DForOutWhenUnconnected=off
  wires:
  Switch1/1 -> Zr/1
  Clock1/1 -> Product/2
  Sine Wave1/1 -> Add/1
  Gain/1 -> Add1/1, Switch/2, Switch1/2
  Switch/1 -> Switch1/3
  Constant1/1 -> Switch/3
  Constant3/1 -> Add1/2
  Constant2/1 -> Product/1
  Product/1 -> Gain/1
  Add1/1 -> Divide/1
  Constant4/1 -> Gain1/1
  Add/1 -> Switch/1
  Constant/1 -> Gain2/1
  Divide/1 -> Sine Wave1/1
  Gain1/1 -> Divide/2
  Constant5/1 -> Switch1/1
  Gain2/1 -> Add/2

== system RL_sus_quarter_sim/road_profile/origin/road_profile/Random ==
  Add : Sum
  Gain : Gain  Gain=2*n0*pi*sqrt(G0*u)
  Gain1 : Gain  Gain=-2*pi*u*n1
  Integrator : Integrator
  WhiteNoise : simulink/Sources/Band-Limited White Noise  Cov=[0.5]  Ts=1/10/u  seed=[24553]
  Zr : Outport  VectorParamsAs1DForOutWhenUnconnected=off
  wires:
  Gain1/1 -> Add/2
  Add/1 -> Integrator/1
  WhiteNoise/1 -> Gain/1
  Integrator/1 -> Zr/1, Gain1/1
  Gain/1 -> Add/1

== system RL_sus_quarter_sim/road_profile/origin/road_profile/Sine ==
  Add : Sum
  Add1 : Sum
  Clock : Clock
  Gain : Gain  Gain=2*pi
  Scope : Scope  NumInputPorts=2
      settings: ActiveDisplayYMinimum=-0.00065  ActiveDisplayYMaximum=0.00585  DataLoggingVariableName=ScopeData2
  Sin : Trigonometry
  Sine Wave : Sin  Commented=on  Amplitude=sine_amp  Bias=sine_amp  Frequency=2*pi*sine_freq  Phase=-pi/2  SampleTime=0
  freq : Gain  Gain=9
  off-set : Constant
  phase : Constant  Value=-pi/2
  sine_amp : Gain  Gain=0.026/9
  Out1 : Outport
  wires:
  sine_amp/1 -> Out1/1, Scope/1
  Sin/1 -> Add/1
  Add/1 -> sine_amp/1
  off-set/1 -> Add/2
  phase/1 -> Add1/2
  Add1/1 -> Sin/1
  Gain/1 -> Add1/1
  freq/1 -> Gain/1
  Clock/1 -> freq/1
  Sine Wave/1 -> Scope/2

== system RL_sus_quarter_sim/road_profile/origin/road_profile/chirp ==
  note: 幅值
  note: 30hz
  note: f=t*0.2
  note: Frequency=0.2*t [Hz]
  note: x=sin(0.2*2pi*t*t)/(0.2*pi*t)
  Clock1 : Clock
  Constant1 : Constant  Value=0.001  SampleTime=0.001
  Constant2 : Constant
  Constant3 : Constant  Value=pi  SampleTime=0.001
  Divide4 : Product  Inputs=*/
  Divide5 : Product  Inputs=**
  Divide6 : Product  Inputs=**
  Divide7 : Product  Inputs=**
  Gain1 : Gain  Gain=0.1
  Gain3 : Gain  Gain=0.2*2/2
  Math Function2 : Math  Operator=square  SignedPower=on
  Switch : Switch  Criteria=u2 > Threshold  SaturateOnIntegerOverflow=off  InputSameDT=off
  Trigonometric Function1 : Trigonometry
  Zr : Outport  VectorParamsAs1DForOutWhenUnconnected=off
  wires:
  Constant2/1 -> Divide4/1
  Switch/1 -> Divide5/1, Math Function2/1
  Divide5/1 -> Divide4/2
  Divide4/1 -> Divide6/1
  Trigonometric Function1/1 -> Divide6/2
  Divide7/1 -> Trigonometric Function1/1
  Math Function2/1 -> Divide7/1
  Constant3/1 -> Gain3/1
  Gain3/1 -> Divide5/2, Divide7/2
  Divide6/1 -> Gain1/1
  Clock1/1 -> Switch/2, Switch/1
  Constant1/1 -> Switch/3
  Gain1/1 -> Zr/1

== system RL_sus_quarter_sim/Quarter_sys/Control/Y_1/ADP_NN/ADP_NN_Controller ==
  xdef : Inport
  vdef : Inport  Port=2
  vs : Inport  Port=3
  as : Inport  Port=4
  au : Inport  Port=5
  xs : Inport  Port=6
  xs_ref : Inport  Port=7
  vs_ref : Inport  Port=8
  Add : Sum
  Add1 : Sum
  Add2 : Sum  Inputs=+++
  Add3 : Sum  Inputs=-+
  Add4 : Sum  Inputs=-+
  Gain : Gain  Gain=10
  Gain2 : Gain  Gain=1000
  Level-2 MATLAB S-Function : M-S-Function  FunctionName=rbf_nn_adp  Parameters=0.05,12
  Mux : Mux  Inputs=10
  Scope{,1..2,4..5} (5 alike) : Scope
      Scope settings: ActiveDisplayYMinimum=-0.71042  ActiveDisplayYMaximum=0.39377
      Scope1 settings: ActiveDisplayYMinimum=-2.44156  ActiveDisplayYMaximum=8.37978  DataLoggingVariableName=ScopeData2
      Scope2 settings: ActiveDisplayYMinimum=-258.82054  ActiveDisplayYMaximum=329.38482  DataLoggingVariableName=ScopeData3
      Scope4 settings: ActiveDisplayYMinimum=-2.6211  ActiveDisplayYMaximum=3.53001  DataLoggingVariableName=ScopeData6
      Scope5 settings: ActiveDisplayYMinimum=-0.12995  ActiveDisplayYMaximum=0.18183  DataLoggingVariableName=ScopeData7
  Scope3 : Scope  NumInputPorts=2
      settings: ActiveDisplayYMinimum=-0.17911  ActiveDisplayYMaximum=0.26143  DataLoggingVariableName=ScopeData4
  cs_est : Gain  Gain=-1500
  ks_est : Gain  Gain=-15000
  m_est : Gain  Gain=300
  Out1 : Outport
  wires:
  vs_ref/1 -> Add4/2, Mux/9
  vdef/1 -> cs_est/1, Mux/2
  Gain/1 -> Add/2
  xs/1 -> Mux/6, Add3/1
  Add3/1 -> Mux/8, Gain/1, Scope3/1  "e"
  Gain2/1 -> Add2/2, Scope2/1
  Add/1 -> Scope/1, Level-2 MATLAB S-Function/2, Gain2/1  "r"
  as/1 -> Mux/4
  xs_ref/1 -> Mux/10, Add3/2
  Mux/1 -> Level-2 MATLAB S-Function/1
  Add4/1 -> Scope3/2, Add/1, Mux/7  "d_e"
  vs/1 -> Mux/3, Add4/1
  Level-2 MATLAB S-Function/1 -> Scope1/1, m_est/1
  xdef/1 -> ks_est/1, Mux/1
  au/1 -> Mux/5
  Add2/1 -> Out1/1
  ks_est/1 -> Add1/1
  cs_est/1 -> Add1/2
  Add1/1 -> Add2/3
  m_est/1 -> Add2/1
  Level-2 MATLAB S-Function/2 -> Scope4/1
  Level-2 MATLAB S-Function/3 -> Scope5/1

== system RL_sus_quarter_sim/Quarter_sys/Control/Y_1/ADP_NN/reference ==
  xs : Inport
  vs : Inport  Port=2
  constant : Subsystem  VariantControl=zero
  skyhook_virtual : Subsystem  VariantControl=skyhook_virtual
  xs_ref : Outport
  vs_ref : Outport  Port=2

== system RL_sus_quarter_sim/Quarter_sys/Control/Y_1/Freq_imp/Low_with_Alpha ==
  v_def : Inport
  a_def : Inport  Port=2
  Ideal Force Sensor : fl_lib/Mechanical/Mechanical Sensors/Ideal Force Sensor
  Ideal Translational Velocity Source : fl_lib/Mechanical/Mechanical Sources/Ideal Translational Velocity Source
  Mechanical Translational Reference : fl_lib/Mechanical/Translational Elements/Mechanical Translational Reference
  Mechanical Translational Reference1 : fl_lib/Mechanical/Translational Elements/Mechanical Translational Reference
  PS-Simulink Converter : nesl_utility/PS-Simulink Converter  PhysicalDomain=network_engine_domain  SubClassName=ps_output  LeftPortType=input  RightPortType=output  PseudoPeriodic=off  Frequencies=[]  VectorFormat=inherit  Unit=inherit  AffineConversion=off
  Simulink-PS Converter : nesl_utility/Simulink-PS Converter  PhysicalDomain=network_engine_domain  SubClassName=ps_input  LeftPortType=input  RightPortType=output  PseudoPeriodic=off  Frequencies=[]  NoiseDistribution=none  NoiseParameters=[]  Unit=1  AffineConversion=off  FilteringAndDerivatives=provide  SimscapeFilterOrder=1  InputFilterTimeConstant=0.001  UdotUserProvided=1
  Solver Configuration : nesl_utility/Solver Configuration  PhysicalDomain=network_engine_domain  SubClassName=solver  LeftPortType=input  RightPortType=generic  Tones=[]  Harmonics=[]  SimulateNoise=off  Profile=off  UseLocalSampling=off  EnableSwitchedLinearOptims=on  FrequencyDomain=off  UseCCode=off  RelTol=0.001  AbsTol=0.001  MinStep=1e-09  ToWorkspace=off  RevertToSquareIcSolve=off  NumHomotopyIterations=100  PhasorMode=off  PhasorModeNumHarmonics=1  ConsistencySolver=NEWTON_XTOL_AFTER_FTOL  IndexReductionMethod=DerivativeReplacement  DoDC=off  ResidualTolerance=1e-09  ConsistencyTolSource=GLOBAL  ConsistencyAbsTol=0.001  ConsistencyRelTol=0.001  ConsistencyTolFactor=0.001  UseLocalSolver=off  LocalSolverChoice=NE_BACKWARD_EULER_ADVANCER  ResolveIndetEquations=on  FunctionEvalNumThread=1  LocalSolverSampleTime=0.001  DoFixedCost=off  MaxNonlinIter=3  MaxModeIter=2  ComputeImpulses=off  ImpulseIterations=2  LinearAlgebra=auto  LinearAlgebraNumThread=0  EquationFormulation=NE_TIME_EF  DelaysMemoryBudget=1024  AutomaticFiltering=on  FilteringTimeConstant=0.001  PartitionStorageMethod=AS_NEEDED  PartitionMemoryBudget=1024  PartitionMethod=ROBUST  MultibodyUseLocalSolver=off  MultibodyLocalSolverChoice=ODE1  MultibodyLocalSolverSampleTime=0.001
  Subsystem : Subsystem  Variant=on  VariantControlMode=label  VariantControl=Subsystem  LabelModeActiveChoice=p1_k5
  F : Outport
  wires:
  v_def/1 -> Simulink-PS Converter/1
  PS-Simulink Converter/1 -> F/1
  a_def/1 -> Simulink-PS Converter/2
  connections:
  Subsystem/LConn1 -- Ideal Translational Velocity Source/RConn2
  PS-Simulink Converter/LConn1 -- Ideal Force Sensor/RConn2
  Simulink-PS Converter/RConn1 -- Ideal Translational Velocity Source/RConn1
  Subsystem/RConn1 -- Ideal Force Sensor/LConn1
  Ideal Translational Velocity Source/LConn1 -- Solver Configuration/RConn1 -- Mechanical Translational Reference1/LConn1
  Ideal Force Sensor/RConn1 -- Mechanical Translational Reference/LConn1

== system RL_sus_quarter_sim/Quarter_sys/Control/Y_1/Freq_imp/high_with_Alpha ==
  v_def : Inport
  a_def : Inport  Port=2
  Ideal Force Sensor : fl_lib/Mechanical/Mechanical Sensors/Ideal Force Sensor
  Ideal Translational Velocity Source : fl_lib/Mechanical/Mechanical Sources/Ideal Translational Velocity Source
  Mechanical Translational Reference : fl_lib/Mechanical/Translational Elements/Mechanical Translational Reference
  Mechanical Translational Reference1 : fl_lib/Mechanical/Translational Elements/Mechanical Translational Reference
  PS-Simulink Converter : nesl_utility/PS-Simulink Converter  PhysicalDomain=network_engine_domain  SubClassName=ps_output  LeftPortType=input  RightPortType=output  PseudoPeriodic=off  Frequencies=[]  VectorFormat=inherit  Unit=inherit  AffineConversion=off
  Simulink-PS Converter : nesl_utility/Simulink-PS Converter  PhysicalDomain=network_engine_domain  SubClassName=ps_input  LeftPortType=input  RightPortType=output  PseudoPeriodic=off  Frequencies=[]  NoiseDistribution=none  NoiseParameters=[]  Unit=1  AffineConversion=off  FilteringAndDerivatives=provide  SimscapeFilterOrder=1  InputFilterTimeConstant=0.001  UdotUserProvided=1
  Solver Configuration : nesl_utility/Solver Configuration  PhysicalDomain=network_engine_domain  SubClassName=solver  LeftPortType=input  RightPortType=generic  Tones=[]  Harmonics=[]  SimulateNoise=off  Profile=off  UseLocalSampling=off  EnableSwitchedLinearOptims=on  FrequencyDomain=off  UseCCode=off  RelTol=0.001  AbsTol=0.001  MinStep=1e-09  ToWorkspace=off  RevertToSquareIcSolve=off  NumHomotopyIterations=100  PhasorMode=off  PhasorModeNumHarmonics=1  ConsistencySolver=NEWTON_XTOL_AFTER_FTOL  IndexReductionMethod=DerivativeReplacement  DoDC=off  ResidualTolerance=1e-09  ConsistencyTolSource=GLOBAL  ConsistencyAbsTol=0.001  ConsistencyRelTol=0.001  ConsistencyTolFactor=0.001  UseLocalSolver=off  LocalSolverChoice=NE_BACKWARD_EULER_ADVANCER  ResolveIndetEquations=on  FunctionEvalNumThread=1  LocalSolverSampleTime=0.001  DoFixedCost=off  MaxNonlinIter=3  MaxModeIter=2  ComputeImpulses=off  ImpulseIterations=2  LinearAlgebra=auto  LinearAlgebraNumThread=0  EquationFormulation=NE_TIME_EF  DelaysMemoryBudget=1024  AutomaticFiltering=on  FilteringTimeConstant=0.001  PartitionStorageMethod=AS_NEEDED  PartitionMemoryBudget=1024  PartitionMethod=ROBUST  MultibodyUseLocalSolver=off  MultibodyLocalSolverChoice=ODE1  MultibodyLocalSolverSampleTime=0.001
  Subsystem : Subsystem  Variant=on  VariantControlMode=label  VariantControl=Subsystem  LabelModeActiveChoice=p1_k1
  F : Outport
  wires:
  a_def/1 -> Simulink-PS Converter/2
  PS-Simulink Converter/1 -> F/1
  v_def/1 -> Simulink-PS Converter/1
  connections:
  Ideal Force Sensor/RConn1 -- Mechanical Translational Reference/LConn1
  Solver Configuration/RConn1 -- Ideal Translational Velocity Source/LConn1 -- Mechanical Translational Reference1/LConn1
  Subsystem/RConn1 -- Ideal Force Sensor/LConn1
  Simulink-PS Converter/RConn1 -- Ideal Translational Velocity Source/RConn1
  PS-Simulink Converter/LConn1 -- Ideal Force Sensor/RConn2
  Subsystem/LConn1 -- Ideal Translational Velocity Source/RConn2

== system RL_sus_quarter_sim/Quarter_sys/Control/Y_1/Freq_imp1/Low_with_Alpha ==
  v_def : Inport
  a_def : Inport  Port=2
  Ideal Force Sensor : fl_lib/Mechanical/Mechanical Sensors/Ideal Force Sensor
  Ideal Translational Velocity Source : fl_lib/Mechanical/Mechanical Sources/Ideal Translational Velocity Source
  Mechanical Translational Reference : fl_lib/Mechanical/Translational Elements/Mechanical Translational Reference
  Mechanical Translational Reference1 : fl_lib/Mechanical/Translational Elements/Mechanical Translational Reference
  PS-Simulink Converter : nesl_utility/PS-Simulink Converter  PhysicalDomain=network_engine_domain  SubClassName=ps_output  LeftPortType=input  RightPortType=output  PseudoPeriodic=off  Frequencies=[]  VectorFormat=inherit  Unit=inherit  AffineConversion=off
  Simulink-PS Converter : nesl_utility/Simulink-PS Converter  PhysicalDomain=network_engine_domain  SubClassName=ps_input  LeftPortType=input  RightPortType=output  PseudoPeriodic=off  Frequencies=[]  NoiseDistribution=none  NoiseParameters=[]  Unit=1  AffineConversion=off  FilteringAndDerivatives=provide  SimscapeFilterOrder=1  InputFilterTimeConstant=0.001  UdotUserProvided=1
  Solver Configuration : nesl_utility/Solver Configuration  PhysicalDomain=network_engine_domain  SubClassName=solver  LeftPortType=input  RightPortType=generic  Tones=[]  Harmonics=[]  SimulateNoise=off  Profile=off  UseLocalSampling=off  EnableSwitchedLinearOptims=on  FrequencyDomain=off  UseCCode=off  RelTol=0.001  AbsTol=0.001  MinStep=1e-09  ToWorkspace=off  RevertToSquareIcSolve=off  NumHomotopyIterations=100  PhasorMode=off  PhasorModeNumHarmonics=1  ConsistencySolver=NEWTON_XTOL_AFTER_FTOL  IndexReductionMethod=DerivativeReplacement  DoDC=off  ResidualTolerance=1e-09  ConsistencyTolSource=GLOBAL  ConsistencyAbsTol=0.001  ConsistencyRelTol=0.001  ConsistencyTolFactor=0.001  UseLocalSolver=off  LocalSolverChoice=NE_BACKWARD_EULER_ADVANCER  ResolveIndetEquations=on  FunctionEvalNumThread=1  LocalSolverSampleTime=0.001  DoFixedCost=off  MaxNonlinIter=3  MaxModeIter=2  ComputeImpulses=off  ImpulseIterations=2  LinearAlgebra=auto  LinearAlgebraNumThread=0  EquationFormulation=NE_TIME_EF  DelaysMemoryBudget=1024  AutomaticFiltering=on  FilteringTimeConstant=0.001  PartitionStorageMethod=AS_NEEDED  PartitionMemoryBudget=1024  PartitionMethod=ROBUST  MultibodyUseLocalSolver=off  MultibodyLocalSolverChoice=ODE1  MultibodyLocalSolverSampleTime=0.001
  Subsystem : Subsystem  Variant=on  VariantControlMode=label  VariantControl=Subsystem  LabelModeActiveChoice=p1_k1
  F : Outport
  wires:
  a_def/1 -> Simulink-PS Converter/2
  PS-Simulink Converter/1 -> F/1
  v_def/1 -> Simulink-PS Converter/1
  connections:
  Ideal Force Sensor/RConn1 -- Mechanical Translational Reference/LConn1
  Mechanical Translational Reference1/LConn1 -- Solver Configuration/RConn1 -- Ideal Translational Velocity Source/LConn1
  Subsystem/RConn1 -- Ideal Force Sensor/LConn1
  Simulink-PS Converter/RConn1 -- Ideal Translational Velocity Source/RConn1
  PS-Simulink Converter/LConn1 -- Ideal Force Sensor/RConn2
  Subsystem/LConn1 -- Ideal Translational Velocity Source/RConn2

== system RL_sus_quarter_sim/Quarter_sys/Control/Y_1/Freq_imp1/Subsystem ==
  vs : Inport
  au : Inport  Port=2
  alpha1 : Inport  Port=3
  alpha2 : Inport  Port=4
  2nd_FS : Subsystem
  Chart : Stateflow chart  TreatAsAtomicUnit=on
  Constant : Constant
  FS1 : Subsystem
  Scope : Scope
      settings: ActiveDisplayYMinimum=1.96975  ActiveDisplayYMaximum=3.01644  DataLoggingVariableName=ScopeData10
  Scope1 : Scope
      settings: ActiveDisplayYMinimum=-8.71775  ActiveDisplayYMaximum=7.25476  DataLoggingVariableName=ScopeData13
  Select : Outport
  wires:
  vs/1 -> FS1/1(vs), 2nd_FS/1(vs)
  FS1/1(FS2) -> ?
  au/1 -> FS1/2(au), 2nd_FS/2(au)
  2nd_FS/1(FS2) -> Scope1/1, Chart/2(FS_2)
  Chart/1(Select) -> Select/1, Scope/1
  alpha2/1 -> 2nd_FS/3(alpha)
  alpha1/1 -> FS1/3(alpha)
  Constant/1 -> Chart/1(FS_1)

== system RL_sus_quarter_sim/Quarter_sys/Control/Y_1/Freq_imp1/high_with_Alpha ==
  v_def : Inport
  a_def : Inport  Port=2
  Ideal Force Sensor : fl_lib/Mechanical/Mechanical Sensors/Ideal Force Sensor
  Ideal Translational Velocity Source : fl_lib/Mechanical/Mechanical Sources/Ideal Translational Velocity Source
  Mechanical Translational Reference : fl_lib/Mechanical/Translational Elements/Mechanical Translational Reference
  Mechanical Translational Reference1 : fl_lib/Mechanical/Translational Elements/Mechanical Translational Reference
  PS-Simulink Converter : nesl_utility/PS-Simulink Converter  PhysicalDomain=network_engine_domain  SubClassName=ps_output  LeftPortType=input  RightPortType=output  PseudoPeriodic=off  Frequencies=[]  VectorFormat=inherit  Unit=inherit  AffineConversion=off
  Simulink-PS Converter : nesl_utility/Simulink-PS Converter  PhysicalDomain=network_engine_domain  SubClassName=ps_input  LeftPortType=input  RightPortType=output  PseudoPeriodic=off  Frequencies=[]  NoiseDistribution=none  NoiseParameters=[]  Unit=1  AffineConversion=off  FilteringAndDerivatives=provide  SimscapeFilterOrder=1  InputFilterTimeConstant=0.001  UdotUserProvided=1
  Solver Configuration : nesl_utility/Solver Configuration  PhysicalDomain=network_engine_domain  SubClassName=solver  LeftPortType=input  RightPortType=generic  Tones=[]  Harmonics=[]  SimulateNoise=off  Profile=off  UseLocalSampling=off  EnableSwitchedLinearOptims=on  FrequencyDomain=off  UseCCode=off  RelTol=0.001  AbsTol=0.001  MinStep=1e-09  ToWorkspace=off  RevertToSquareIcSolve=off  NumHomotopyIterations=100  PhasorMode=off  PhasorModeNumHarmonics=1  ConsistencySolver=NEWTON_XTOL_AFTER_FTOL  IndexReductionMethod=DerivativeReplacement  DoDC=off  ResidualTolerance=1e-09  ConsistencyTolSource=GLOBAL  ConsistencyAbsTol=0.001  ConsistencyRelTol=0.001  ConsistencyTolFactor=0.001  UseLocalSolver=off  LocalSolverChoice=NE_BACKWARD_EULER_ADVANCER  ResolveIndetEquations=on  FunctionEvalNumThread=1  LocalSolverSampleTime=0.001  DoFixedCost=off  MaxNonlinIter=3  MaxModeIter=2  ComputeImpulses=off  ImpulseIterations=2  LinearAlgebra=auto  LinearAlgebraNumThread=0  EquationFormulation=NE_TIME_EF  DelaysMemoryBudget=1024  AutomaticFiltering=on  FilteringTimeConstant=0.001  PartitionStorageMethod=AS_NEEDED  PartitionMemoryBudget=1024  PartitionMethod=ROBUST  MultibodyUseLocalSolver=off  MultibodyLocalSolverChoice=ODE1  MultibodyLocalSolverSampleTime=0.001
  Subsystem : Subsystem  Variant=on  VariantControlMode=label  VariantControl=Subsystem  LabelModeActiveChoice=p1_k5
  F : Outport
  wires:
  v_def/1 -> Simulink-PS Converter/1
  PS-Simulink Converter/1 -> F/1
  a_def/1 -> Simulink-PS Converter/2
  connections:
  Subsystem/LConn1 -- Ideal Translational Velocity Source/RConn2
  PS-Simulink Converter/LConn1 -- Ideal Force Sensor/RConn2
  Simulink-PS Converter/RConn1 -- Ideal Translational Velocity Source/RConn1
  Subsystem/RConn1 -- Ideal Force Sensor/LConn1
  Ideal Translational Velocity Source/LConn1 -- Solver Configuration/RConn1 -- Mechanical Translational Reference1/LConn1
  Ideal Force Sensor/RConn1 -- Mechanical Translational Reference/LConn1

== system RL_sus_quarter_sim/Quarter_sys/Control/Y_1/IFEKF FDC/ADD ==
  v_def : Inport
  a_s : Inport  Port=2
  Add : Sum
  Constant : Constant  Value=-1
  Constant1 : Constant
  Delta_C : Gain  Gain=500
  Gain1 : Gain  Gain=-1
  Lmbada_C : Constant  Value=1000
  Product : Product
  Product2 : Product
  Switch : Switch  Criteria=u2 > Threshold  SaturateOnIntegerOverflow=off  InputSameDT=off
  Out1 : Outport
  wires:
  Lmbada_C/1 -> Add/2
  Delta_C/1 -> Add/1
  Constant1/1 -> Switch/1
  Constant/1 -> Switch/3
  Product2/1 -> Gain1/1
  v_def/1 -> Product2/1, Product/1
  a_s/1 -> Product/2
  Switch/1 -> Delta_C/1
  Add/1 -> Product2/2
  Product/1 -> Switch/2
  Gain1/1 -> Out1/1
